simulink subsystem "StreetLaneSegment1x1_BUS_asSubsystem"  (R2021a)
settings: Solver=VariableStepAuto  StartTime=0.0  StopTime=10.0  RelTol=1e-3
libraries: StreetLanesLibrary x1
settings Model: Creator=phill  LastModifiedBy=phill

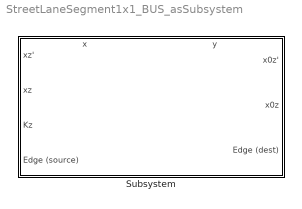
== system StreetLaneSegment1x1_BUS_asSubsystem ==
  Subsystem : Subsystem  mask{Kz=0, Tz=0}
      mask prompts: Kz "Kz (Capacity - How many cars fit into this cell)"; Tz "Tz (Nominal travel time for vehicles traveling unobstructed through the cell)"
      mask help:
      | This Block models a single Street-Lane capable of holding / transducing cars (or at least "car volume units") as a cell. This 1x1 version It is connected to a single source edge (over which it can receive cars from a preceeding cell) and a single destination edge (over which it can lose cars to the succeeding cell).  It has a capacity (how many volume-units of cars can be present on the segment at a given time) and a nominal travel time (how long cars would need to travel through it unobstructed). The outputs are:
      |
      | x0z  : how many cars (in car volume units) are "at the end of the cell" (and thus visible for the destination-edge  or the following cell).  The value can only rise if more cars flow in (mind the delay Tz!) than flow out - for instance if a traffic light blocks the exit.
      | x0z' : the rate of change for the number of cars "at the end of the cell". Will be positive when more cars arrive than drive out, and negative when more cars leave it.
      | xz    : how many cars are in the cell in total (both the ones who just entered and have not reached the end yet, as well as the ones at the end)
      | xz'   : how many cars are flowing into- (positive sign) or out of (negative) the cell per time
      | yz    : the internal flow - how many cars pass into the "endpart" of a cell. It is delayed by Tz compared to the incoming flow y_incoming, so any cars that enter a cell will only "appear visible" at the end of it after that time Tz.
      | yin : the total flow of cars into the cell
      | yout : the total flow of cars out of the cell
      settings: PortSchema="{\"entries\":[{\"content\":{\"sides\":[{\"content\":{\"connectorIds\":[\"Out5\",\"Out6\",\"Out7\",\"In1\"]},\"type\":\"ConnectorPlacement.EquallySpacedRectSide\",\"uuid\":\"fa7777a8-ec1a-439f-ac9e-e0ed45345ec6\"},{\"content\":{\"connectorIds\":[\"Out1\",\"Out2\",\"In2\"],\"side\":\"RIGHT\"},\"type\":\"ConnectorPlacement.EquallySpacedRectSide\",\"uuid\":\"1d8f22c6-fff9-419e-a471-d80b757471c2\"},{\"content\":{\"connectorIds\":[\"Out3\",\"Out4\"],\"side\":\"TOP\"},\"type\":\"ConnectorPlacement.EquallySpacedRectSide\",\"uuid\":\"5603a277-4601-4f1d-99e7-cf6c913c8902\"}]},\"type\":\"ConnectorPlacement.EquallySpacedConnector\",\"uuid\":\"948237b2-05cb-41b3-a7da-b6feef56487f\"}],\"packageUris\":[\"http://schema.mathworks.com/mf0/Connector/R2020b\"],\"version\":\"1.0\"}"
      mask Display:
      | image('$imagefile'); % Use "Edit Image" on toolstrip to change.
      | %image('$imagefile');
      | disp('Street Lane Segment 1x1 \n\n');
      | disp(['Kz = ', get_param(gcb,'Kz'), ' | Tz = ', get_param(gcb, 'Tz')])

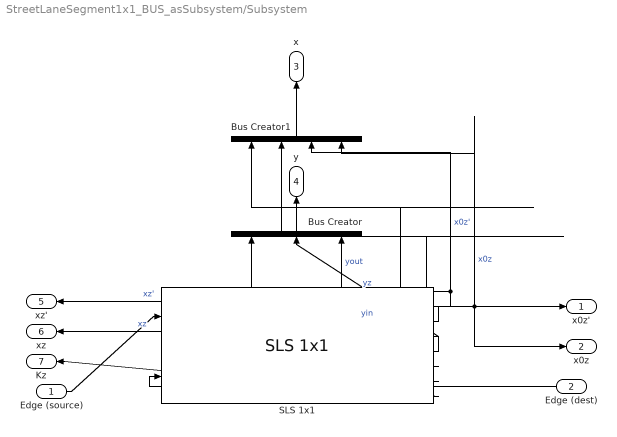
== system StreetLaneSegment1x1_BUS_asSubsystem/Subsystem ==
  Edge (source) : Inport
  Edge (dest) : Inport  Port=2
  Bus Creator : BusCreator  Inputs=3
  Bus Creator1 : BusCreator  Inputs=4
  SLS 1x1 : StreetLanesLibrary/SLS 1x1  Kz=0  Tz=0
  x0z' : Outport
  x0z : Outport  Port=2
  x : Outport  Port=3
  y : Outport  Port=4
  xz' : Outport  Port=5
  xz : Outport  Port=6
  Kz : Outport  Port=7
  wires:
  SLS 1x1/8 -> Kz/1
  SLS 1x1/5 -> Bus Creator/3  "yout"
  SLS 1x1/1 -> x0z'/1, Bus Creator1/3  "x0z'"
  SLS 1x1/2 -> x0z/1, Bus Creator1/4  "x0z"
  SLS 1x1/7 -> xz/1, Bus Creator1/1  "xz"
  SLS 1x1/6 -> xz'/1, Bus Creator1/2  "xz'"
  Bus Creator/1 -> y/1
  SLS 1x1/3 -> Bus Creator/1  "yin"
  Bus Creator1/1 -> x/1
  SLS 1x1/4 -> Bus Creator/2  "yz"
  Edge (source)/1 -> SLS 1x1/1
  Edge (dest)/1 -> SLS 1x1/2
